simulink model "mcb_pmsm_foc_hall"  (R2025b)
settings: Solver=FixedStepDiscrete  StartTime=0.0  StopTime=8  RelTol=1e-3  EnableMultiTasking=on
InitFcn:
  | mcb_pmsm_foc_hall_AK45_10_KV75_data;
model workspace (MAT data in the model file):
  encoderResolution = 2000
  hallOffset = '0.5'
  indexOffset = 850
  polePairs = '4'
values from neighbouring files (symbols this model uses):
  dataType = 'single'    [mcb_pmsm_foc_hall_AK45_10_KV75_data.m]
  inverter = mcb.updateInverterParameters(pmsm,inverter,target)    [mcb_pmsm_foc_hall_AK45_10_KV75_data.m]
  PI_params = mcb.getPIControllerParameters(pmsm,inverter,PU_System,T_pwm,Ts,Ts_speed)    [mcb_pmsm_foc_hall_AK45_10_KV75_data.m]
  pmsm = struct()    [getMotorParameters.m]    (also in mcb_pmsm_foc_hall_AK45_10_KV75_data.m = getMotorParameters('AK45_36_KV80'))
  PU_System = mcb.getPUSystemParameters(pmsm,inverter)    [mcb_pmsm_foc_hall_AK45_10_KV75_data.m]
  T_pwm = 1/PWM_frequency    (= 5e-05)    [mcb_pmsm_foc_hall_AK45_10_KV75_data.m]
  target = mcb.getProcessorParameters('F28379D',PWM_frequency)    [mcb_pmsm_foc_hall_AK45_10_KV75_data.m]
  Ts = T_pwm    (= 5e-05)    [mcb_pmsm_foc_hall_AK45_10_KV75_data.m]
  Ts_motor = T_pwm/2    (= 2.5e-05)    [mcb_pmsm_foc_hall_AK45_10_KV75_data.m]
  Ts_simulink = T_pwm/2    (= 2.5e-05)    [mcb_pmsm_foc_hall_AK45_10_KV75_data.m]
  Ts_speed = 10*Ts    (= 0.0005)    [mcb_pmsm_foc_hall_AK45_10_KV75_data.m]
undefined symbols (not defined in the file or in its folder): bit, Down, GPTRIP1SEL, GPTRIP2SEL, TZ1, TZ2, Up
libraries: simulink x27, idelinklib_common x8, c280xlib x8, mcbpositiondecoderlib x7, c2802xlib x7, mcbcontrolslib x6, svdschedulerlib x5, mcbeeMathTransformLib x3, slpidlib x3, c2837xDlib x3, svdutilitieslib x1, mcbplantlib x1
(part 3 of 3)

== system mcb_pmsm_foc_hall/Current Control/Input Scaling/Read_Sensor (codegen)/Convert ADC value to PU ==
  Iab_meas_ADC : Inport
  Add : Sum  Inputs=-+
  Data Store Read : DataStoreRead  DataStoreName=IaOffset  IndexOptions=Index vector (dialog)  Indices=1  OutputSizes=1
  Data Store Read1 : DataStoreRead  DataStoreName=IbOffset  IndexOptions=Index vector (dialog)  Indices=1  OutputSizes=1
  Data Type Conversion : DataTypeConversion  OutDataTypeStr=int32  ConvertRealWorld=Stored Integer (SI)  SaturateOnIntegerOverflow=off  RndMeth=Floor
  Data_Type : Subsystem  Variant=on
  Inverting / Non-inverting Current measurement amplifieer : Gain  Gain=inverter.invertingAmp  RndMeth=Simplest  OutDataTypeStr=Inherit: Same as input
  Mux : Mux  Inputs=2
  Iab_meas_PU : Outport
  wires:
  Add/1 -> Data_Type/1(In1)
  Mux/1 -> Add/1
  Data Type Conversion/1 -> Add/2
  Iab_meas_ADC/1 -> Data Type Conversion/1
  Data Store Read/1 -> Mux/1
  Data Store Read1/1 -> Mux/2
  Data_Type/1(Iab_meas_PU) -> Inverting / Non-inverting Current measurement amplifieer/1
  Inverting / Non-inverting Current measurement amplifieer/1 -> Iab_meas_PU/1

== system mcb_pmsm_foc_hall/Current Control/Input Scaling/Read_Sensor (sim)/Convert ADC value to PU ==
  Iab_meas_ADC : Inport
  0A in ADC counts : Constant  Value=[inverter.CtSensAOffset inverter.CtSensBOffset]  OutDataTypeStr=uint16  SampleTime=-1
  Add : Sum  Inputs=-+
  Data Type Conversion : DataTypeConversion  OutDataTypeStr=int32  ConvertRealWorld=Stored Integer (SI)  SaturateOnIntegerOverflow=off  RndMeth=Floor
  Data_Type : Subsystem  Variant=on
  Inverting / Non-inverting Current measurement amplifieer : Gain  Gain=inverter.invertingAmp  RndMeth=Simplest  OutDataTypeStr=Inherit: Same as input
  Iab_meas_PU : Outport  InitialOutput=0  VectorParamsAs1DForOutWhenUnconnected=off
  wires:
  Data Type Conversion/1 -> Add/2
  Iab_meas_ADC/1 -> Data Type Conversion/1
  0A in ADC counts/1 -> Add/1
  Data_Type/1(Iab_meas_PU) -> Inverting / Non-inverting Current measurement amplifieer/1
  Add/1 -> Data_Type/1(In1)
  Inverting / Non-inverting Current measurement amplifieer/1 -> Iab_meas_PU/1

== system mcb_pmsm_foc_hall/Current Control/Input Scaling/Read_Sensor (sim)/Convert meas angle to PU ==
  Pos_Sim : Inport
  Data Type Conversion1 : DataTypeConversion  OutDataTypeStr=dataType  RndMeth=Simplest  SaturateOnIntegerOverflow=off
  IIR Filter : mcbcontrolslib/IIR Filter  VariantControl=Low Pass Filter  VariantSelect=Low-pass  FilterConstantInputType=Specify via dialog  Filter_constant=0.01  InitialOutput=Specify via dialog  InitialOutputValue=0  ExternalReset=none  advancedSettings=off  Ts=50e-6  cutOff_freq=32.1525
  Mechanical to Electrical Position : mcbpositiondecoderlib/Mechanical to Electrical Position  PolePairsInputType=Specify via dialog  NrPP=pmsm.p  selectedRange=Per unit  MechOfstInputType=Specify via dialog  mechOffsetIn=0  maxAngleIn=1  InputDataType=dataType  VariantSelect=floating-point
  Speed Measurement : mcbpositiondecoderlib/Speed Measurement  DiscreteStepInput=off  LastDiscreteStepInput=off  PositionUnit=Per unit  PositionScalingDatatype=uint32  SpeedCalculationMode=Time interval for speed calculation  TempSpeedCalculationMode=Time interval for speed calculation  SampleTimeAsync=Ts  MaximumApplicationSpeed=6000  SpeedResolution=5e-6  DelayLength=20  MaximumMeasurableSpeed=28571.4286  MeasurableSpeedResolution=1.397e-05  SpeedUnit=Per unit based on dialog  TempSpeedUnit=RPM  PerUnitSpeed=PU_System.N_base  SpeedDataType=dataType
  Theta : Outport
  Speed : Outport  Port=2
  wires:
  Pos_Sim/1 -> Speed Measurement/1, Mechanical to Electrical Position/1
  Mechanical to Electrical Position/1 -> Data Type Conversion1/1
  Data Type Conversion1/1 -> Theta/1
  Speed Measurement/1 -> IIR Filter/1
  IIR Filter/1 -> Speed/1

== system mcb_pmsm_foc_hall/Current Control/SCI_Tx/Code Generation/Data_Conditioning_Tx ==
  In1 : Inport
  Data_Type_Fixed_Point : Subsystem  VariantControl=~isequal(dataType,'single')
  Data_Type_Float : Subsystem  VariantControl=isequal(dataType, 'single')
  Data_Log : Outport

== system mcb_pmsm_foc_hall/Current Control/SCI_Tx/Code Generation/Data_Logging ==
  note: Fast Serial Data Monitoring (32-bit)
  Data_Log : Inport
  Counter Limited : simulink/Sources/Counter Limited  uplimit=600-1  tsamp=-1
  Data : Subsystem  TreatAsAtomicUnit=on
  End : Subsystem  TreatAsAtomicUnit=on
  If : If  IfExpression=u1 == 0  ElseIfExpressions=u1 == 599
  Merge : Merge  Inputs=3
  Merge1 : Merge  Inputs=3
  Mux : Mux  Inputs=2
  Start : Subsystem  TreatAsAtomicUnit=on
  Width : Width  OutDataTypeMode=All ports same datatype  DataType=uint16
  SCI_Tx : Outport
  wires:
  If/3 -> Data/Action
  Data/1(Data_out) -> Merge/3
  Width/1 -> Data/2(Data_width), Start/2(Data_width), End/2(Data_width)
  Merge/1 -> Mux/1  "SCI_Tx_Data"
  Counter Limited/1 -> If/1
  Start/2(Iteration) -> Merge1/1
  Start/1(Data_out) -> Merge/1
  If/2 -> End/Action
  Merge1/1 -> Mux/2  "SCI_Tx_Iteration"
  If/1 -> Start/Action
  End/1(Data_out) -> Merge/2
  End/2(Iteration) -> Merge1/2
  Data/2(Iteration) -> Merge1/3
  Mux/1 -> SCI_Tx/1
  Data_Log/1 -> Width/1, Start/1(Data), End/1(Data), Data/1(Data)

== system mcb_pmsm_foc_hall/Current Control/SCI_Tx/Code Generation/While Iterator Subsystem ==
  Data : Inport
  Iteration : Inport  Port=2
  Add : Sum  Inputs=+-  OutDataTypeStr=Inherit: Same as first input
  Index Vector : MultiPortSwitch  Inputs=1  SaturateOnIntegerOverflow=off  InputSameDT=off
  SCI Transmit : c280xlib/SCI Transmit  sciModule=A  dataHead=''  dataTail=''  frameSize=1  blockingMode=on  outputStatus=off
  While Iterator : WhileIterator  MaxIters=-1  WhileBlockType=do-while  ShowIterationPort=on  OutputDataType=int16
  wires:
  While Iterator/1 -> Add/2, Index Vector/1
  Data/1 -> Index Vector/2
  Index Vector/1 -> SCI Transmit/1
  Add/1 -> While Iterator/1
  Iteration/1 -> Add/1

== system mcb_pmsm_foc_hall/Hall Sensor A/HallValidity/CodeGen/Read Halls ==
  note: GPIO 54
  note: GPIO 55
  note: GPIO 57
  Bitwise Operator2 : simulink/Logic and Bit Operations/Bitwise Operator  logicop=OR  UseBitMask=off  NumInputPorts=3  BitMask=hex2dec('07000000')  BitMaskRealWorld=Stored Integer
  Hall_A : simulink/Logic and Bit Operations/Bitwise Operator  logicop=AND  UseBitMask=on  BitMask=hex2dec('00400000')  BitMaskRealWorld=Stored Integer
  Hall_B : simulink/Logic and Bit Operations/Bitwise Operator  logicop=AND  UseBitMask=on  BitMask=hex2dec('00800000')  BitMaskRealWorld=Stored Integer
  Hall_C : simulink/Logic and Bit Operations/Bitwise Operator  logicop=AND  UseBitMask=on  BitMask=hex2dec('02000000')  BitMaskRealWorld=Stored Integer
  Read GPIO DAT register : idelinklib_common/Memory Copy  copyFrom=Specified source code symbol  copyFromAddressSource=Specify via dialog  copyFromAddress=hex2dec('6FC1')  copyFromSrcCode=&GpioDataRegs.GPBDAT.all  dataTypeFrom=uint32  dataDimensionFrom=1  useOffsetFrom=off  offsetFromSrc=Specify via dialog  offsetFrom=0  strideFrom=1  copyTo=Output port  copyToAddressSource=Specify via dialog  copyToAddress=hex2dec('00002000')  copyToSrcCode=GpioDataRegs.GPADAT.bit.GPIO24  dataTypeTo=uint32  useOffsetTo=off  offsetToSrc=Specify via dialog  offsetTo=0  strideTo=1  sampleTime=-1  useInitValue=off  initValueSrc=Specify constant value  initValue=1  initValueSrcCode=myInitValueVariable  useAsMask=off  maskOperator=bitwise AND  useTermValue=off  termValue=1  isRealtimeEnabled=off  emitCCBeforeWrite=off  CCBeforeWrite=/* Custom Code Before Write*/  emitCCAfterWrite=off  CCAfterWrite=/* Custom Code After Write*/
  Shift Arithmetic : ArithShift  BitShiftNumber=23
  Shift Arithmetic1 : ArithShift  BitShiftNumber=22
  Shift Arithmetic2 : ArithShift  BitShiftNumber=22
  Halls : Outport
  wires:
  Hall_C/1 -> Shift Arithmetic/1
  Hall_A/1 -> Shift Arithmetic2/1
  Read GPIO DAT register/1 -> Hall_C/1, Hall_A/1, Hall_B/1
  Hall_B/1 -> Shift Arithmetic1/1
  Bitwise Operator2/1 -> Halls/1
  Shift Arithmetic/1 -> Bitwise Operator2/1
  Shift Arithmetic1/1 -> Bitwise Operator2/2
  Shift Arithmetic2/1 -> Bitwise Operator2/3

== system mcb_pmsm_foc_hall/Hall Sensor B/HallValidity/CodeGen/Read Halls ==
  note: GPIO 54
  note: GPIO 55
  note: GPIO 57
  Bitwise Operator2 : simulink/Logic and Bit Operations/Bitwise Operator  logicop=OR  UseBitMask=off  NumInputPorts=3  BitMask=hex2dec('07000000')  BitMaskRealWorld=Stored Integer
  Hall_A : simulink/Logic and Bit Operations/Bitwise Operator  logicop=AND  UseBitMask=on  BitMask=hex2dec('00400000')  BitMaskRealWorld=Stored Integer
  Hall_B : simulink/Logic and Bit Operations/Bitwise Operator  logicop=AND  UseBitMask=on  BitMask=hex2dec('00800000')  BitMaskRealWorld=Stored Integer
  Hall_C : simulink/Logic and Bit Operations/Bitwise Operator  logicop=AND  UseBitMask=on  BitMask=hex2dec('02000000')  BitMaskRealWorld=Stored Integer
  Read GPIO DAT register : idelinklib_common/Memory Copy  copyFrom=Specified source code symbol  copyFromAddressSource=Specify via dialog  copyFromAddress=hex2dec('6FC1')  copyFromSrcCode=&GpioDataRegs.GPBDAT.all  dataTypeFrom=uint32  dataDimensionFrom=1  useOffsetFrom=off  offsetFromSrc=Specify via dialog  offsetFrom=0  strideFrom=1  copyTo=Output port  copyToAddressSource=Specify via dialog  copyToAddress=hex2dec('00002000')  copyToSrcCode=GpioDataRegs.GPADAT.bit.GPIO24  dataTypeTo=uint32  useOffsetTo=off  offsetToSrc=Specify via dialog  offsetTo=0  strideTo=1  sampleTime=-1  useInitValue=off  initValueSrc=Specify constant value  initValue=1  initValueSrcCode=myInitValueVariable  useAsMask=off  maskOperator=bitwise AND  useTermValue=off  termValue=1  isRealtimeEnabled=off  emitCCBeforeWrite=off  CCBeforeWrite=/* Custom Code Before Write*/  emitCCAfterWrite=off  CCAfterWrite=/* Custom Code After Write*/
  Shift Arithmetic : ArithShift  BitShiftNumber=23
  Shift Arithmetic1 : ArithShift  BitShiftNumber=22
  Shift Arithmetic2 : ArithShift  BitShiftNumber=22
  Halls : Outport
  wires:
  Hall_C/1 -> Shift Arithmetic/1
  Hall_A/1 -> Shift Arithmetic2/1
  Read GPIO DAT register/1 -> Hall_C/1, Hall_A/1, Hall_B/1
  Hall_B/1 -> Shift Arithmetic1/1
  Bitwise Operator2/1 -> Halls/1
  Shift Arithmetic/1 -> Bitwise Operator2/1
  Shift Arithmetic1/1 -> Bitwise Operator2/2
  Shift Arithmetic2/1 -> Bitwise Operator2/3

== system mcb_pmsm_foc_hall/Hall Sensor C/HallValidity/CodeGen/Read Halls ==
  note: GPIO 54
  note: GPIO 55
  note: GPIO 57
  Bitwise Operator2 : simulink/Logic and Bit Operations/Bitwise Operator  logicop=OR  UseBitMask=off  NumInputPorts=3  BitMask=hex2dec('07000000')  BitMaskRealWorld=Stored Integer
  Hall_A : simulink/Logic and Bit Operations/Bitwise Operator  logicop=AND  UseBitMask=on  BitMask=hex2dec('00400000')  BitMaskRealWorld=Stored Integer
  Hall_B : simulink/Logic and Bit Operations/Bitwise Operator  logicop=AND  UseBitMask=on  BitMask=hex2dec('00800000')  BitMaskRealWorld=Stored Integer
  Hall_C : simulink/Logic and Bit Operations/Bitwise Operator  logicop=AND  UseBitMask=on  BitMask=hex2dec('02000000')  BitMaskRealWorld=Stored Integer
  Read GPIO DAT register : idelinklib_common/Memory Copy  copyFrom=Specified source code symbol  copyFromAddressSource=Specify via dialog  copyFromAddress=hex2dec('6FC1')  copyFromSrcCode=&GpioDataRegs.GPBDAT.all  dataTypeFrom=uint32  dataDimensionFrom=1  useOffsetFrom=off  offsetFromSrc=Specify via dialog  offsetFrom=0  strideFrom=1  copyTo=Output port  copyToAddressSource=Specify via dialog  copyToAddress=hex2dec('00002000')  copyToSrcCode=GpioDataRegs.GPADAT.bit.GPIO24  dataTypeTo=uint32  useOffsetTo=off  offsetToSrc=Specify via dialog  offsetTo=0  strideTo=1  sampleTime=-1  useInitValue=off  initValueSrc=Specify constant value  initValue=1  initValueSrcCode=myInitValueVariable  useAsMask=off  maskOperator=bitwise AND  useTermValue=off  termValue=1  isRealtimeEnabled=off  emitCCBeforeWrite=off  CCBeforeWrite=/* Custom Code Before Write*/  emitCCAfterWrite=off  CCAfterWrite=/* Custom Code After Write*/
  Shift Arithmetic : ArithShift  BitShiftNumber=23
  Shift Arithmetic1 : ArithShift  BitShiftNumber=22
  Shift Arithmetic2 : ArithShift  BitShiftNumber=22
  Halls : Outport
  wires:
  Hall_C/1 -> Shift Arithmetic/1
  Hall_A/1 -> Shift Arithmetic2/1
  Read GPIO DAT register/1 -> Hall_C/1, Hall_A/1, Hall_B/1
  Hall_B/1 -> Shift Arithmetic1/1
  Bitwise Operator2/1 -> Halls/1
  Shift Arithmetic/1 -> Bitwise Operator2/1
  Shift Arithmetic1/1 -> Bitwise Operator2/2
  Shift Arithmetic2/1 -> Bitwise Operator2/3

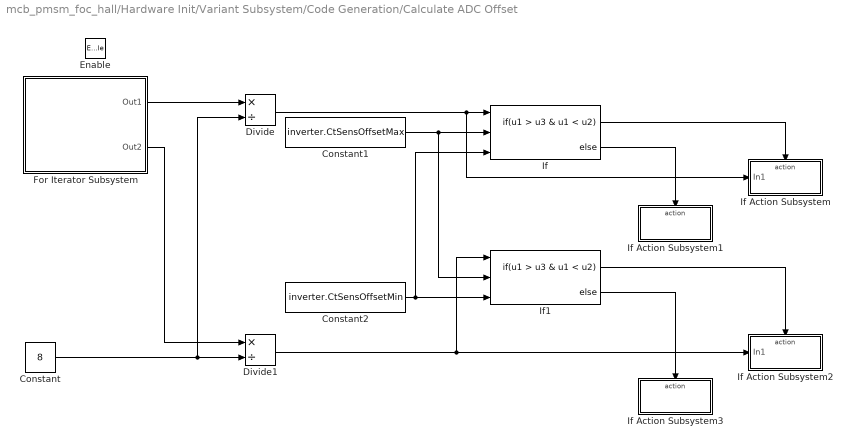
== system mcb_pmsm_foc_hall/Hardware Init/Variant Subsystem/Code Generation/Calculate ADC Offset  ==
  Enable : EnablePort
  Constant : Constant  Value=8
  Constant1 : Constant  Value=inverter.CtSensOffsetMax  OutDataTypeStr=Inherit: Inherit via back propagation
  Constant2 : Constant  Value=inverter.CtSensOffsetMin  OutDataTypeStr=Inherit: Inherit via back propagation
  Divide : Product  Inputs=*/  OutDataTypeStr=uint16
  Divide1 : Product  Inputs=*/  OutDataTypeStr=uint16
  For Iterator Subsystem : Subsystem  TreatAsAtomicUnit=on
  If : If  NumInputs=3  IfExpression=u1 > u3 & u1 < u2
  If Action Subsystem : Subsystem  TreatAsAtomicUnit=on
  If Action Subsystem1 : Subsystem  TreatAsAtomicUnit=on
  If Action Subsystem2 : Subsystem  TreatAsAtomicUnit=on
  If Action Subsystem3 : Subsystem  TreatAsAtomicUnit=on
  If1 : If  NumInputs=3  IfExpression=u1 > u3 & u1 < u2
  wires:
  For Iterator Subsystem/1(Out1) -> Divide/1
  If1/2 -> If Action Subsystem3/Action
  If1/1 -> If Action Subsystem2/Action
  If/2 -> If Action Subsystem1/Action
  For Iterator Subsystem/2(Out2) -> Divide1/1
  If/1 -> If Action Subsystem/Action
  Constant2/1 -> If/3, If1/3
  Constant1/1 -> If/2, If1/2
  Divide1/1 -> If1/1, If Action Subsystem2/1(In1)
  Constant/1 -> Divide/2, Divide1/2
  Divide/1 -> If Action Subsystem/1(In1), If/1

== system mcb_pmsm_foc_hall/Hardware Init/Variant Subsystem/Code Generation/DRV Enable ==
  In : Inport
  ADC Gain Setting : Subsystem
  Constant : Constant  OutDataTypeStr=Inherit: Inherit via back propagation
  Constant1 : Constant  Value=inverter.EnableLogic
  DRV830x Enable : c2837xDlib/Digital Output  GPIO_Number=GPIO120~GPIO127  GPIO_Bit0=off  GPIO_BIT0_Toggle=off  GPIO_Bit1=off  GPIO_BIT1_Toggle=off  GPIO_Bit2=off  GPIO_BIT2_Toggle=off  GPIO_Bit3=off  GPIO_BIT3_Toggle=off  GPIO_Bit4=on  GPIO_BIT4_Toggle=off  GPIO_Bit5=off  GPIO_BIT5_Toggle=off  GPIO_Bit6=off  GPIO_BIT6_Toggle=off  GPIO_Bit7=off  GPIO_BIT7_Toggle=off
  NOT : Logic  Operator=NOT  IconShape=distinctive  AllPortsSameDT=off  OutDataTypeStr=boolean
  Switch : Switch  Criteria=u2 > Threshold  SaturateOnIntegerOverflow=off  InputSameDT=off
  wires:
  NOT/1 -> Switch/3  "Active low logic for inverter enable"
  Switch/1 -> DRV830x Enable/1
  Constant/1 -> Switch/1, NOT/1  "Active high logic for inverter enable"
  Constant1/1 -> ADC Gain Setting/Enable, Switch/2
  In/1 -> ADC Gain Setting/1(In1)

== system mcb_pmsm_foc_hall/Hardware Init/Variant Subsystem/Code Generation/Default ADC Offset ==
  Enable : EnablePort
  Constant : Constant  Value=inverter.CtSensAOffset  OutDataTypeStr=Inherit: Inherit via back propagation
  Constant1 : Constant  Value=inverter.CtSensBOffset  OutDataTypeStr=Inherit: Inherit via back propagation
  Data Store Write1 : DataStoreWrite  DataStoreName=IaOffset  IndexOptions=Index vector (dialog)  Indices=1  OutputSizes=1
  Data Store Write2 : DataStoreWrite  DataStoreName=IbOffset  IndexOptions=Index vector (dialog)  Indices=1  OutputSizes=1
  wires:
  Constant/1 -> Data Store Write1/1
  Constant1/1 -> Data Store Write2/1

== system mcb_pmsm_foc_hall/Serial Receive/SCI_Rx/Code Generation/Data_Type_Fixed_Point ==
  SCI Receive : c280xlib/SCI Receive  sciModule=A  dataHead=''  headerCheckMaxCount=16  dataTail=''  dataType=uint32  dataLenOptions=Length via dialog  dataDim=2  maxDataLength=1  initValue=0  errOption=Output the last received value  errValue=0  sampleTime=-1  blockingMode=on  timeOut=0.00875  outputStatus=off
  Data : Outport
  wires:
  SCI Receive/1 -> Data/1

== system mcb_pmsm_foc_hall/Serial Receive/SCI_Rx/Code Generation/Data_Type_Float ==
  SCI Receive : c280xlib/SCI Receive  sciModule=A  dataHead=''  headerCheckMaxCount=16  dataTail=''  dataType=single  dataLenOptions=Length via dialog  dataDim=2  maxDataLength=1  initValue=0  errOption=Output the last received value  errValue=0  sampleTime=-1  blockingMode=on  timeOut=0.00875  outputStatus=off
  Data : Outport
  wires:
  SCI Receive/1 -> Data/1

== system mcb_pmsm_foc_hall/Serial Receive/SCI_Rx/Simulation/Data_Conditioning_Tx ==
  In1 : Inport
  In2 : Inport  Port=2
  Data_Type_Fixed_Point : Subsystem  VariantControl=~isequal(dataType, 'single')
  Data_Type_Float : Subsystem  VariantControl=isequal(dataType, 'single')
  Data : Outport

== system mcb_pmsm_foc_hall/Serial Receive/SCI_Rx/Simulation/Parse ==
  Enable_PWM : Inport
  Debug_signals : Inport  Port=2
  Bitwise Operator : simulink/Logic and Bit Operations/Bitwise Operator  logicop=AND  UseBitMask=on  BitMask=hex2dec('0001')  BitMaskRealWorld=Stored Integer
  Bitwise Operator1 : simulink/Logic and Bit Operations/Bitwise Operator  logicop=AND  UseBitMask=on  BitMask=hex2dec('00F0')  BitMaskRealWorld=Stored Integer
  Shift Arithmetic1 : ArithShift  BitShiftNumber=-4
  Sum : Sum
  Data : Outport
  wires:
  Bitwise Operator/1 -> Sum/1
  Debug_signals/1 -> Shift Arithmetic1/1
  Sum/1 -> Data/1
  Shift Arithmetic1/1 -> Bitwise Operator1/1
  Enable_PWM/1 -> Bitwise Operator/1
  Bitwise Operator1/1 -> Sum/2

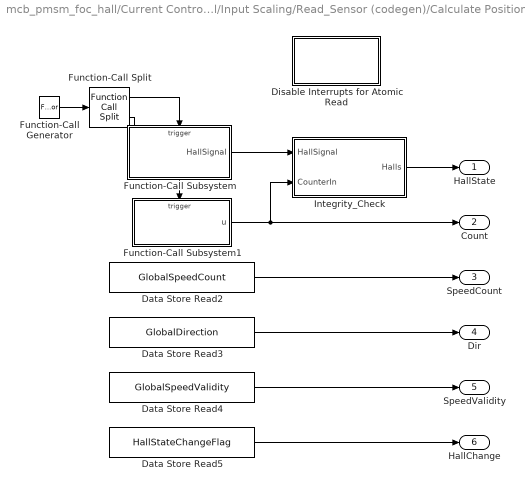
== system mcb_pmsm_foc_hall/Current Control/Input Scaling/Read_Sensor (codegen)/Calculate Position from Hall/Atomic Hall Reading ==
  Data Store Read2 : DataStoreRead  DataStoreName=GlobalSpeedCount  IndexOptions=Index vector (dialog)  Indices=1  OutputSizes=1
  Data Store Read3 : DataStoreRead  DataStoreName=GlobalDirection  IndexOptions=Index vector (dialog)  Indices=1  OutputSizes=1
  Data Store Read4 : DataStoreRead  DataStoreName=GlobalSpeedValidity  IndexOptions=Index vector (dialog)  Indices=1  OutputSizes=1
  Data Store Read5 : DataStoreRead  Priority=1  DataStoreName=HallStateChangeFlag  IndexOptions=Index vector (dialog)  Indices=1  OutputSizes=1
  Disable Interrupts for Atomic Read : Subsystem  mask(System Outputs){ShowInLibBrowser=0}
      mask prompts: ShowInLibBrowser "Simulink:masks:CustCodeMaskParam1_MP"
      settings: CopyFcn=cccopyfcn(gcb)  OpenFcn=ccopenfcn('System Outputs Function')
      mask Help: eval('feval(''rtwprivate'',''rtwhelpview'',''rtw_sys_outputs_block'')');
      mask Display: disp('System\nOutputs');
  Function-Call Generator : FunctionCallGenerator  SampleTime=-1
  Function-Call Split : FunctionCallSplit  NumOutputPorts=2  OutputPortLayout=default
  Function-Call Subsystem : Subsystem  TreatAsAtomicUnit=on
  Function-Call Subsystem1 : Subsystem  TreatAsAtomicUnit=on
  Integrity_Check : Subsystem
  HallState : Outport
  Count : Outport  Port=2
  SpeedCount : Outport  Port=3
  Dir : Outport  Port=4
  SpeedValidity : Outport  Port=5
  HallChange : Outport  Port=6
  wires:
  Data Store Read4/1 -> SpeedValidity/1
  Data Store Read3/1 -> Dir/1
  Data Store Read2/1 -> SpeedCount/1
  Data Store Read5/1 -> HallChange/1
  Function-Call Subsystem1/1(u) -> Integrity_Check/2(CounterIn), Count/1
  Integrity_Check/1(Halls) -> HallState/1
  Function-Call Generator/1 -> Function-Call Split/1
  Function-Call Split/1 -> Function-Call Subsystem/Trigger
  Function-Call Split/2 -> Function-Call Subsystem1/Trigger
  Function-Call Subsystem/1(HallSignal) -> Integrity_Check/1(HallSignal)

== system mcb_pmsm_foc_hall/Current Control/Input Scaling/Read_Sensor (codegen)/Calculate Position from Hall/Subsystem ==
  Input : Inport
  Enable : EnablePort
  Output : Outport
  wires:
  Input/1 -> Output/1

== system mcb_pmsm_foc_hall/Current Control/Input Scaling/Read_Sensor (codegen)/Convert ADC value to PU/Data_Type ==
  In1 : Inport
  Data_Type_Fixed_Point : Subsystem  VariantControl=~isequal(dataType,'single')
  Data_Type_Float : Subsystem  VariantControl=isequal(dataType,'single')
  Iab_meas_PU : Outport

== system mcb_pmsm_foc_hall/Current Control/Input Scaling/Read_Sensor (sim)/Convert ADC value to PU/Data_Type ==
  In1 : Inport
  Data_Type_Fixed_Point : Subsystem  VariantControl=~isequal(dataType,'single')
  Data_Type_Float : Subsystem  VariantControl=isequal(dataType,'single')
  Iab_meas_PU : Outport

== system mcb_pmsm_foc_hall/Current Control/SCI_Tx/Code Generation/Data_Conditioning_Tx/Data_Type_Fixed_Point ==
  In1 : Inport
  Data Type Conversion : DataTypeConversion  OutDataTypeStr=fixdt(1,32,28)  RndMeth=Simplest  SaturateOnIntegerOverflow=off
  Data Type Conversion3 : DataTypeConversion  OutDataTypeStr=uint32  ConvertRealWorld=Stored Integer (SI)  RndMeth=Simplest  SaturateOnIntegerOverflow=off
  Data_Log : Outport
  wires:
  In1/1 -> Data Type Conversion/1
  Data Type Conversion3/1 -> Data_Log/1
  Data Type Conversion/1 -> Data Type Conversion3/1

== system mcb_pmsm_foc_hall/Current Control/SCI_Tx/Code Generation/Data_Conditioning_Tx/Data_Type_Float ==
  In1 : Inport
  Byte Pack : svdutilitieslib/Byte Pack  maskPackedDataType=uint32  datatypes={'single'}  byteAlign=4  blockPlatform=tic2000
  Data_Log : Outport
  wires:
  Byte Pack/1 -> Data_Log/1
  In1/1 -> Byte Pack/1

== system mcb_pmsm_foc_hall/Current Control/SCI_Tx/Code Generation/Data_Logging/Data ==
  Data : Inport
  Data_width : Inport  Port=2
  Action Port : ActionPort
  Dummy : Constant  Value=hex2dec('0000')  OutDataTypeStr=uint32
  Mux : Mux  Inputs=2
  Data_out : Outport  VectorParamsAs1DForOutWhenUnconnected=off
  Iteration : Outport  Port=2  VectorParamsAs1DForOutWhenUnconnected=off
  wires:
  Data_width/1 -> Iteration/1
  Data/1 -> Mux/1
  Dummy/1 -> Mux/2
  Mux/1 -> Data_out/1

== system mcb_pmsm_foc_hall/Current Control/SCI_Tx/Code Generation/Data_Logging/End ==
  Data : Inport
  Data_width : Inport  Port=2
  Action Port : ActionPort
  Bias : Bias  Bias=1  SaturateOnIntegerOverflow=off
  End : Constant  Value=hex2dec('45454545')  OutDataTypeStr=uint32
  Mux : Mux  Inputs=2
  Data_out : Outport  VectorParamsAs1DForOutWhenUnconnected=off
  Iteration : Outport  Port=2  VectorParamsAs1DForOutWhenUnconnected=off
  wires:
  Data/1 -> Mux/1
  Data_width/1 -> Bias/1
  Bias/1 -> Iteration/1
  End/1 -> Mux/2
  Mux/1 -> Data_out/1

== system mcb_pmsm_foc_hall/Current Control/SCI_Tx/Code Generation/Data_Logging/Start ==
  Data : Inport
  Data_width : Inport  Port=2
  Action Port : ActionPort
  Bias : Bias  Bias=1  SaturateOnIntegerOverflow=off
  Mux : Mux  Inputs=2
  Start : Constant  Value=hex2dec('53535353')  OutDataTypeStr=uint32
  Data_out : Outport  VectorParamsAs1DForOutWhenUnconnected=off
  Iteration : Outport  Port=2  VectorParamsAs1DForOutWhenUnconnected=off
  wires:
  Data/1 -> Mux/2
  Data_width/1 -> Bias/1
  Bias/1 -> Iteration/1
  Start/1 -> Mux/1
  Mux/1 -> Data_out/1

== system mcb_pmsm_foc_hall/Hardware Init/Variant Subsystem/Code Generation/Calculate ADC Offset /For Iterator Subsystem ==
  ADC_A_IN0 : c2802xlib/ADC  Priority=20  blkParamProc=C2000_Type4  ADCModule=C  samplingMode=Single sample mode  ADCResolution=12-bit (Single-ended input)  ADC29xResolution=12-bit  ADCMode=Single-ended input  useSOC1=SOC2  useSOC2=SOC0_SOC1  SOCAcquisitionWindow=15  SOCTriggerSource=Software  SOCInterruptTrigger=No ADCINT  Ts=-1  dType=uint16  postInterrupt=off  interruptSel=ADCINT1  ADCINTContinuous=on  endma=off  chdma=1  conv1=ADCINA0  conv2=ADCINA0 and ADCINB0  conv1_Type4=ADCIN2  conv2_Type4=ADCIN0 and ADCIN1
  ADC_B_IN0 : c2802xlib/ADC  Priority=20  blkParamProc=C2000_Type4  ADCModule=B  samplingMode=Single sample mode  ADCResolution=12-bit (Single-ended input)  ADC29xResolution=12-bit  ADCMode=Single-ended input  useSOC1=SOC2  useSOC2=SOC0_SOC1  SOCAcquisitionWindow=15  SOCTriggerSource=Software  SOCInterruptTrigger=No ADCINT  Ts=-1  dType=uint16  postInterrupt=off  interruptSel=ADCINT1  ADCINTContinuous=on  endma=off  chdma=1  conv1=ADCINA0  conv2=ADCINA0 and ADCINB0  conv1_Type4=ADCIN2  conv2_Type4=ADCIN0 and ADCIN1
  For Iterator : ForIterator  IterationLimit=16  IterationVariableDataType=uint16
  If : If  IfExpression=u1 > 8  ShowElse=off
  If Action Subsystem : Subsystem  TreatAsAtomicUnit=on
  Out1 : Outport
  Out2 : Outport  Port=2
  wires:
  For Iterator/1 -> If/1
  ADC_A_IN0/1 -> If Action Subsystem/1(In1)
  ADC_B_IN0/1 -> If Action Subsystem/2(In2)
  If Action Subsystem/1(Out1) -> Out1/1
  If Action Subsystem/2(Out2) -> Out2/1
  If/1 -> If Action Subsystem/Action

== system mcb_pmsm_foc_hall/Hardware Init/Variant Subsystem/Code Generation/Calculate ADC Offset /If Action Subsystem ==
  In1 : Inport
  Action Port : ActionPort
  Data Store Write1 : DataStoreWrite  DataStoreName=IaOffset  IndexOptions=Index vector (dialog)  Indices=1  OutputSizes=1
  wires:
  In1/1 -> Data Store Write1/1

== system mcb_pmsm_foc_hall/Hardware Init/Variant Subsystem/Code Generation/Calculate ADC Offset /If Action Subsystem1 ==
  Action Port : ActionPort
  Constant : Constant  Value=inverter.CtSensAOffset  OutDataTypeStr=Inherit: Inherit via back propagation
  Data Store Write1 : DataStoreWrite  DataStoreName=IaOffset  IndexOptions=Index vector (dialog)  Indices=1  OutputSizes=1
  wires:
  Constant/1 -> Data Store Write1/1

== system mcb_pmsm_foc_hall/Hardware Init/Variant Subsystem/Code Generation/Calculate ADC Offset /If Action Subsystem2 ==
  In1 : Inport
  Action Port : ActionPort
  Data Store Write2 : DataStoreWrite  DataStoreName=IbOffset  IndexOptions=Index vector (dialog)  Indices=1  OutputSizes=1
  wires:
  In1/1 -> Data Store Write2/1

== system mcb_pmsm_foc_hall/Hardware Init/Variant Subsystem/Code Generation/Calculate ADC Offset /If Action Subsystem3 ==
  Action Port : ActionPort
  Constant1 : Constant  Value=inverter.CtSensBOffset  OutDataTypeStr=Inherit: Inherit via back propagation
  Data Store Write2 : DataStoreWrite  DataStoreName=IbOffset  IndexOptions=Index vector (dialog)  Indices=1  OutputSizes=1
  wires:
  Constant1/1 -> Data Store Write2/1

== system mcb_pmsm_foc_hall/Hardware Init/Variant Subsystem/Code Generation/DRV Enable/ADC Gain Setting ==
  In1 : Inport
  Enable : EnablePort
  Demux : Demux  Outputs=2
  Display : Display
      settings: Format=hex (Stored Integer)
  Display1 : Display
      settings: Format=hex (Stored Integer)
  SPI Master Transfer2 : c280xlib/SPI Controller Transfer  SPISelect=SPI_A  ClockPolarity=Rising_edge  ClockPhase=No_delay  SPIModule=uint32(0)  Mode=Master  BusSpeed=uint32(1000000)  FirstBitToTransfer=Most significant bit (MSB)  ClockMode=0  BlockFunction=Transfer  EnableRegisterAddress=off  RegisterAddress=0  OutputDataType=int8  OutputDataLength=1  DataBits=16  UseCustomSSPin=Provided by the SPI peripheral  ActiveLowSSPin=Active low  Pin=61
  SPI Master Transfer3 : c280xlib/SPI Controller Transfer  SPISelect=SPI_A  ClockPolarity=Rising_edge  ClockPhase=No_delay  SPIModule=uint32(0)  Mode=Master  BusSpeed=uint32(1000000)  FirstBitToTransfer=Most significant bit (MSB)  ClockMode=0  BlockFunction=Transfer  EnableRegisterAddress=off  RegisterAddress=0  OutputDataType=int8  OutputDataLength=1  DataBits=16  UseCustomSSPin=Provided by the SPI peripheral  ActiveLowSSPin=Active low  Pin=61
  wires:
  SPI Master Transfer3/1 -> Display1/1
  Demux/1 -> SPI Master Transfer2/1
  SPI Master Transfer2/1 -> Display/1
  Demux/2 -> SPI Master Transfer3/1
  In1/1 -> Demux/1

== system mcb_pmsm_foc_hall/Serial Receive/SCI_Rx/Simulation/Data_Conditioning_Tx/Data_Type_Fixed_Point ==
  In1 : Inport
  In2 : Inport  Port=2
  Data Type Conversion : DataTypeConversion  OutDataTypeStr=fixdt(1,32,28)  RndMeth=Simplest  SaturateOnIntegerOverflow=off
  Data Type Conversion1 : DataTypeConversion  OutDataTypeStr=uint32  RndMeth=Simplest  SaturateOnIntegerOverflow=off
  Data Type Conversion3 : DataTypeConversion  OutDataTypeStr=uint32  ConvertRealWorld=Stored Integer (SI)  RndMeth=Simplest  SaturateOnIntegerOverflow=off
  Mux : Mux  Inputs=2
  Data : Outport
  wires:
  In1/1 -> Data Type Conversion/1
  Data Type Conversion3/1 -> Mux/1
  Data Type Conversion/1 -> Data Type Conversion3/1
  In2/1 -> Data Type Conversion1/1
  Data Type Conversion1/1 -> Mux/2
  Mux/1 -> Data/1

== system mcb_pmsm_foc_hall/Serial Receive/SCI_Rx/Simulation/Data_Conditioning_Tx/Data_Type_Float ==
  In1 : Inport
  In2 : Inport  Port=2
  Data Type Conversion2 : DataTypeConversion  OutDataTypeStr=single  RndMeth=Simplest  SaturateOnIntegerOverflow=off
  Mux : Mux  Inputs=2
  Data : Outport
  wires:
  In1/1 -> Mux/1
  Mux/1 -> Data/1
  In2/1 -> Data Type Conversion2/1
  Data Type Conversion2/1 -> Mux/2

== system mcb_pmsm_foc_hall/Current Control/Input Scaling/Read_Sensor (codegen)/Calculate Position from Hall/Atomic Hall Reading/Disable Interrupts for Atomic Read ==

== system mcb_pmsm_foc_hall/Current Control/Input Scaling/Read_Sensor (codegen)/Calculate Position from Hall/Atomic Hall Reading/Function-Call Subsystem ==
  function : TriggerPort  TriggerType=function-call  VariantControl=Variant
  Read Halls : Subsystem  mask(Hall sensor reader){sample_time=-1}
      mask prompts: sample_time "Sample time:"
      mask help:
      | This block outputs the state of the 3 hall sensors placed on GPIO54, 55 and 57 of LaunchXL-F28379D board.
      |
      | 0 --> GPIO57 = 0, GPIO55 = 0, GPIO54 = 0
      | 1 --> GPIO57 = 0, GPIO55 = 0, GPIO54 = 1
      | 2 --> GPIO57 = 0, GPIO55 = 1, GPIO54 = 0
      | 3 --> GPIO57 = 0, GPIO55 = 1, GPIO54 = 1
      | 4 --> GPIO57 = 1, GPIO55 = 0, GPIO54 = 0
      | 5 --> GPIO57 = 1, GPIO55 = 0, GPIO54 = 1
      | 6 --> GPIO57 = 1, GPIO55 = 1, GPIO54 = 0
      | 7 --> GPIO57 = 1, GPIO55 = 1, GPIO54 = 1
  HallSignal : Outport
  wires:
  Read Halls/1(Halls) -> HallSignal/1

== system mcb_pmsm_foc_hall/Current Control/Input Scaling/Read_Sensor (codegen)/Calculate Position from Hall/Atomic Hall Reading/Function-Call Subsystem1 ==
  function : TriggerPort  TriggerType=function-call  VariantControl=Variant
  Memory Copy : idelinklib_common/Memory Copy  copyFrom=Specified source code symbol  copyFromAddressSource=Specify via dialog  copyFromAddress=hex2dec('00001000')  copyFromSrcCode=&ECap1Regs.TSCTR  dataTypeFrom=uint32  dataDimensionFrom=1  useOffsetFrom=off  offsetFromSrc=Specify via dialog  offsetFrom=0  strideFrom=1  copyTo=Output port  copyToAddressSource=Specify via dialog  copyToAddress=hex2dec('00002000')  copyToSrcCode=myVariableDst  dataTypeTo=uint32  useOffsetTo=off  offsetToSrc=Specify via dialog  offsetTo=0  strideTo=1  sampleTime=-1  useInitValue=off  initValueSrc=Specify constant value  initValue=1  initValueSrcCode=myInitValueVariable  useAsMask=off  maskOperator=bitwise AND  useTermValue=off  termValue=1  isRealtimeEnabled=off  emitCCBeforeWrite=off  CCBeforeWrite=/* Custom Code Before Write*/  emitCCAfterWrite=off  CCAfterWrite=/* Custom Code After Write*/
  Memory Copy1 : idelinklib_common/Memory Copy  copyFrom=Specified source code symbol  copyFromAddressSource=Specify via dialog  copyFromAddress=hex2dec('00001000')  copyFromSrcCode=&ECap2Regs.TSCTR  dataTypeFrom=uint32  dataDimensionFrom=1  useOffsetFrom=off  offsetFromSrc=Specify via dialog  offsetFrom=0  strideFrom=1  copyTo=Output port  copyToAddressSource=Specify via dialog  copyToAddress=hex2dec('00002000')  copyToSrcCode=myVariableDst  dataTypeTo=uint32  useOffsetTo=off  offsetToSrc=Specify via dialog  offsetTo=0  strideTo=1  sampleTime=-1  useInitValue=off  initValueSrc=Specify constant value  initValue=1  initValueSrcCode=myInitValueVariable  useAsMask=off  maskOperator=bitwise AND  useTermValue=off  termValue=1  isRealtimeEnabled=off  emitCCBeforeWrite=off  CCBeforeWrite=/* Custom Code Before Write*/  emitCCAfterWrite=off  CCAfterWrite=/* Custom Code After Write*/
  Memory Copy2 : idelinklib_common/Memory Copy  copyFrom=Specified source code symbol  copyFromAddressSource=Specify via dialog  copyFromAddress=hex2dec('00001000')  copyFromSrcCode=&ECap3Regs.TSCTR  dataTypeFrom=uint32  dataDimensionFrom=1  useOffsetFrom=off  offsetFromSrc=Specify via dialog  offsetFrom=0  strideFrom=1  copyTo=Output port  copyToAddressSource=Specify via dialog  copyToAddress=hex2dec('00002000')  copyToSrcCode=myVariableDst  dataTypeTo=uint32  useOffsetTo=off  offsetToSrc=Specify via dialog  offsetTo=0  strideTo=1  sampleTime=-1  useInitValue=off  initValueSrc=Specify constant value  initValue=1  initValueSrcCode=myInitValueVariable  useAsMask=off  maskOperator=bitwise AND  useTermValue=off  termValue=1  isRealtimeEnabled=off  emitCCBeforeWrite=off  CCBeforeWrite=/* Custom Code Before Write*/  emitCCAfterWrite=off  CCAfterWrite=/* Custom Code After Write*/
  Min : MinMax  Inputs=3
  u : Outport
  wires:
  Min/1 -> u/1
  Memory Copy2/1 -> Min/3
  Memory Copy/1 -> Min/1
  Memory Copy1/1 -> Min/2

== system mcb_pmsm_foc_hall/Current Control/Input Scaling/Read_Sensor (codegen)/Calculate Position from Hall/Atomic Hall Reading/Integrity_Check ==
  HallSignal : Inport
  CounterIn : Inport  Port=2
  Compare To Constant : simulink/Logic and Bit Operations/Compare To Constant  relop=<  const=Ts*target.CPU_frequency*0.5  OutDataTypeStr=uint8
  If : If  IfExpression=u1 == 0
  Merge : Merge
  NOT : Logic  IconShape=distinctive  AllPortsSameDT=off  OutDataTypeStr=boolean
  No_Integrity_issue : Subsystem  TreatAsAtomicUnit=on
  Refresh_Halls : Subsystem  TreatAsAtomicUnit=on
  Relational Operator : RelationalOperator  Operator===  OutDataTypeStr=boolean  RndMeth=Simplest  InputSameDT=off
  Unit Delay : UnitDelay  SampleTime=-1  HasFrameUpgradeWarning=on
  Halls : Outport
  wires:
  Refresh_Halls/1(Out1) -> Merge/2
  HallSignal/1 -> Relational Operator/1, No_Integrity_issue/1(Counter), Unit Delay/1
  If/2 -> Refresh_Halls/Action
  Merge/1 -> Halls/1
  No_Integrity_issue/1(Out1) -> Merge/1
  If/1 -> No_Integrity_issue/Action
  CounterIn/1 -> Compare To Constant/1
  Compare To Constant/1 -> NOT/2
  Relational Operator/1 -> NOT/1
  NOT/1 -> If/1
  Unit Delay/1 -> Relational Operator/2

== system mcb_pmsm_foc_hall/Current Control/Input Scaling/Read_Sensor (codegen)/Convert ADC value to PU/Data_Type/Data_Type_Fixed_Point ==
  In1 : Inport
  Data Type Conversion : DataTypeConversion  OutDataTypeStr=fixdt(1,32,17)  ConvertRealWorld=Stored Integer (SI)  RndMeth=Simplest  SaturateOnIntegerOverflow=off
  Data Type Conversion1 : DataTypeConversion  OutDataTypeStr=dataType  RndMeth=Simplest  SaturateOnIntegerOverflow=off
  Q17 per unit conversion : ArithShift  BitShiftNumber=-6
  Iab_meas_PU : Outport
  wires:
  In1/1 -> Q17 per unit conversion/1
  Data Type Conversion1/1 -> Iab_meas_PU/1
  Data Type Conversion/1 -> Data Type Conversion1/1
  Q17 per unit conversion/1 -> Data Type Conversion/1

== system mcb_pmsm_foc_hall/Current Control/Input Scaling/Read_Sensor (codegen)/Convert ADC value to PU/Data_Type/Data_Type_Float ==
  In1 : Inport
  Get ADC Voltage : Gain  Gain=target.ADC_Vref /target.ADC_MaxCount  OutDataTypeStr=dataType  RndMeth=Simplest
  Get Currents : Gain  Gain=1/inverter.ISenseVoltPerAmp  RndMeth=Simplest  OutDataTypeStr=Inherit: Same as input
  PU_Conversion : Gain  Gain=1/PU_System.I_base  RndMeth=Simplest  OutDataTypeStr=Inherit: Same as input
  Iab_meas_PU : Outport
  wires:
  Get Currents/1 -> PU_Conversion/1
  PU_Conversion/1 -> Iab_meas_PU/1
  Get ADC Voltage/1 -> Get Currents/1
  In1/1 -> Get ADC Voltage/1

== system mcb_pmsm_foc_hall/Current Control/Input Scaling/Read_Sensor (sim)/Convert ADC value to PU/Data_Type/Data_Type_Fixed_Point ==
  In1 : Inport
  Data Type Conversion : DataTypeConversion  OutDataTypeStr=fixdt(1,32,17)  ConvertRealWorld=Stored Integer (SI)  RndMeth=Simplest  SaturateOnIntegerOverflow=off
  Data Type Conversion1 : DataTypeConversion  OutDataTypeStr=dataType  RndMeth=Simplest  SaturateOnIntegerOverflow=off
  Q17 per unit conversion : ArithShift  BitShiftNumber=-6
  Iab_meas_PU : Outport
  wires:
  In1/1 -> Q17 per unit conversion/1
  Data Type Conversion1/1 -> Iab_meas_PU/1
  Data Type Conversion/1 -> Data Type Conversion1/1
  Q17 per unit conversion/1 -> Data Type Conversion/1

== system mcb_pmsm_foc_hall/Current Control/Input Scaling/Read_Sensor (sim)/Convert ADC value to PU/Data_Type/Data_Type_Float ==
  In1 : Inport
  Current Sense Gain : Gain  Gain=PU_System.I_base/1.65  RndMeth=Simplest  OutDataTypeStr=Inherit: Same as input
  Get_ADC_Volt : Gain  Gain=1.65/2048  OutDataTypeStr=dataType  RndMeth=Simplest
  PU_Conversion : Gain  Gain=1/PU_System.I_base  RndMeth=Simplest  OutDataTypeStr=Inherit: Same as input
  Iab_meas_PU : Outport
  wires:
  Current Sense Gain/1 -> PU_Conversion/1
  In1/1 -> Get_ADC_Volt/1
  Get_ADC_Volt/1 -> Current Sense Gain/1
  PU_Conversion/1 -> Iab_meas_PU/1

== system mcb_pmsm_foc_hall/Hardware Init/Variant Subsystem/Code Generation/Calculate ADC Offset /For Iterator Subsystem/If Action Subsystem ==
  In1 : Inport
  In2 : Inport  Port=2
  Action Port : ActionPort
  Memory : Memory  InheritSampleTime=on
  Memory1 : Memory  InheritSampleTime=on
  Sum : Sum
  Sum1 : Sum
  Out1 : Outport
  Out2 : Outport  Port=2
  wires:
  In1/1 -> Sum/1
  Sum/1 -> Out1/1, Memory/1
  In2/1 -> Sum1/1
  Memory/1 -> Sum/2
  Sum1/1 -> Out2/1, Memory1/1
  Memory1/1 -> Sum1/2

== system mcb_pmsm_foc_hall/Current Control/Input Scaling/Read_Sensor (codegen)/Calculate Position from Hall/Atomic Hall Reading/Function-Call Subsystem/Read Halls ==
  note: GPIO 54
  note: GPIO 55
  note: GPIO 57
  Bitwise Operator2 : simulink/Logic and Bit Operations/Bitwise Operator  logicop=OR  UseBitMask=off  NumInputPorts=3  BitMask=hex2dec('07000000')  BitMaskRealWorld=Stored Integer
  Hall_A : simulink/Logic and Bit Operations/Bitwise Operator  logicop=AND  UseBitMask=on  BitMask=hex2dec('00400000')  BitMaskRealWorld=Stored Integer
  Hall_B : simulink/Logic and Bit Operations/Bitwise Operator  logicop=AND  UseBitMask=on  BitMask=hex2dec('00800000')  BitMaskRealWorld=Stored Integer
  Hall_C : simulink/Logic and Bit Operations/Bitwise Operator  logicop=AND  UseBitMask=on  BitMask=hex2dec('02000000')  BitMaskRealWorld=Stored Integer
  Read GPIO DAT register : idelinklib_common/Memory Copy  copyFrom=Specified source code symbol  copyFromAddressSource=Specify via dialog  copyFromAddress=hex2dec('6FC1')  copyFromSrcCode=&GpioDataRegs.GPBDAT.all  dataTypeFrom=uint32  dataDimensionFrom=1  useOffsetFrom=off  offsetFromSrc=Specify via dialog  offsetFrom=0  strideFrom=1  copyTo=Output port  copyToAddressSource=Specify via dialog  copyToAddress=hex2dec('00002000')  copyToSrcCode=GpioDataRegs.GPADAT.bit.GPIO24  dataTypeTo=uint32  useOffsetTo=off  offsetToSrc=Specify via dialog  offsetTo=0  strideTo=1  sampleTime=-1  useInitValue=off  initValueSrc=Specify constant value  initValue=1  initValueSrcCode=myInitValueVariable  useAsMask=off  maskOperator=bitwise AND  useTermValue=off  termValue=1  isRealtimeEnabled=off  emitCCBeforeWrite=off  CCBeforeWrite=/* Custom Code Before Write*/  emitCCAfterWrite=off  CCAfterWrite=/* Custom Code After Write*/
  Shift Arithmetic : ArithShift  BitShiftNumber=23
  Shift Arithmetic1 : ArithShift  BitShiftNumber=22
  Shift Arithmetic2 : ArithShift  BitShiftNumber=22
  Halls : Outport
  wires:
  Hall_C/1 -> Shift Arithmetic/1
  Hall_A/1 -> Shift Arithmetic2/1
  Read GPIO DAT register/1 -> Hall_C/1, Hall_A/1, Hall_B/1
  Hall_B/1 -> Shift Arithmetic1/1
  Bitwise Operator2/1 -> Halls/1
  Shift Arithmetic/1 -> Bitwise Operator2/1
  Shift Arithmetic1/1 -> Bitwise Operator2/2
  Shift Arithmetic2/1 -> Bitwise Operator2/3

== system mcb_pmsm_foc_hall/Current Control/Input Scaling/Read_Sensor (codegen)/Calculate Position from Hall/Atomic Hall Reading/Integrity_Check/No_Integrity_issue ==
  Counter : Inport
  Action Port : ActionPort  ActionPortLabel=if(u1 == 0)
  Out1 : Outport
  wires:
  Counter/1 -> Out1/1

== system mcb_pmsm_foc_hall/Current Control/Input Scaling/Read_Sensor (codegen)/Calculate Position from Hall/Atomic Hall Reading/Integrity_Check/Refresh_Halls ==
  Action Port : ActionPort  ActionPortLabel=else
  Read Halls : Subsystem  mask(Hall sensor reader){sample_time=-1}
      mask prompts: sample_time "Sample time:"
      mask help:
      | This block outputs the state of the 3 hall sensors placed on GPIO54, 55 and 57 of LaunchXL-F28379D board.
      |
      | 0 --> GPIO57 = 0, GPIO55 = 0, GPIO54 = 0
      | 1 --> GPIO57 = 0, GPIO55 = 0, GPIO54 = 1
      | 2 --> GPIO57 = 0, GPIO55 = 1, GPIO54 = 0
      | 3 --> GPIO57 = 0, GPIO55 = 1, GPIO54 = 1
      | 4 --> GPIO57 = 1, GPIO55 = 0, GPIO54 = 0
      | 5 --> GPIO57 = 1, GPIO55 = 0, GPIO54 = 1
      | 6 --> GPIO57 = 1, GPIO55 = 1, GPIO54 = 0
      | 7 --> GPIO57 = 1, GPIO55 = 1, GPIO54 = 1
  Out1 : Outport
  wires:
  Read Halls/1(Halls) -> Out1/1

== system mcb_pmsm_foc_hall/Current Control/Input Scaling/Read_Sensor (codegen)/Calculate Position from Hall/Atomic Hall Reading/Integrity_Check/Refresh_Halls/Read Halls ==
  note: GPIO 54
  note: GPIO 55
  note: GPIO 57
  Bitwise Operator2 : simulink/Logic and Bit Operations/Bitwise Operator  logicop=OR  UseBitMask=off  NumInputPorts=3  BitMask=hex2dec('07000000')  BitMaskRealWorld=Stored Integer
  Hall_A : simulink/Logic and Bit Operations/Bitwise Operator  logicop=AND  UseBitMask=on  BitMask=hex2dec('00400000')  BitMaskRealWorld=Stored Integer
  Hall_B : simulink/Logic and Bit Operations/Bitwise Operator  logicop=AND  UseBitMask=on  BitMask=hex2dec('00800000')  BitMaskRealWorld=Stored Integer
  Hall_C : simulink/Logic and Bit Operations/Bitwise Operator  logicop=AND  UseBitMask=on  BitMask=hex2dec('02000000')  BitMaskRealWorld=Stored Integer
  Read GPIO DAT register : idelinklib_common/Memory Copy  copyFrom=Specified source code symbol  copyFromAddressSource=Specify via dialog  copyFromAddress=hex2dec('6FC1')  copyFromSrcCode=&GpioDataRegs.GPBDAT.all  dataTypeFrom=uint32  dataDimensionFrom=1  useOffsetFrom=off  offsetFromSrc=Specify via dialog  offsetFrom=0  strideFrom=1  copyTo=Output port  copyToAddressSource=Specify via dialog  copyToAddress=hex2dec('00002000')  copyToSrcCode=GpioDataRegs.GPADAT.bit.GPIO24  dataTypeTo=uint32  useOffsetTo=off  offsetToSrc=Specify via dialog  offsetTo=0  strideTo=1  sampleTime=-1  useInitValue=off  initValueSrc=Specify constant value  initValue=1  initValueSrcCode=myInitValueVariable  useAsMask=off  maskOperator=bitwise AND  useTermValue=off  termValue=1  isRealtimeEnabled=off  emitCCBeforeWrite=off  CCBeforeWrite=/* Custom Code Before Write*/  emitCCAfterWrite=off  CCAfterWrite=/* Custom Code After Write*/
  Shift Arithmetic : ArithShift  BitShiftNumber=23
  Shift Arithmetic1 : ArithShift  BitShiftNumber=22
  Shift Arithmetic2 : ArithShift  BitShiftNumber=22
  Halls : Outport
  wires:
  Hall_C/1 -> Shift Arithmetic/1
  Hall_A/1 -> Shift Arithmetic2/1
  Read GPIO DAT register/1 -> Hall_C/1, Hall_A/1, Hall_B/1
  Hall_B/1 -> Shift Arithmetic1/1
  Bitwise Operator2/1 -> Halls/1
  Shift Arithmetic/1 -> Bitwise Operator2/1
  Shift Arithmetic1/1 -> Bitwise Operator2/2
  Shift Arithmetic2/1 -> Bitwise Operator2/3
